simulink model "HW6_Q3_2slx_2021a"  (R2021a)
settings: Solver=VariableStepAuto  StartTime=0.0  StopTime=15.0  RelTol=1e-3
settings Model: Creator=USER  LastModifiedBy=USER
settings DebuggingCC: UnconnectedInputMsg=none  UnconnectedOutputMsg=none  UnconnectedLineMsg=none
settings ModelReferenceCC: EnableRefExpFcnMdlSchedulingChecks=off
settings RTWCC: Description=Generic Real-Time Target  DLArmComputeVersion=20.02.1

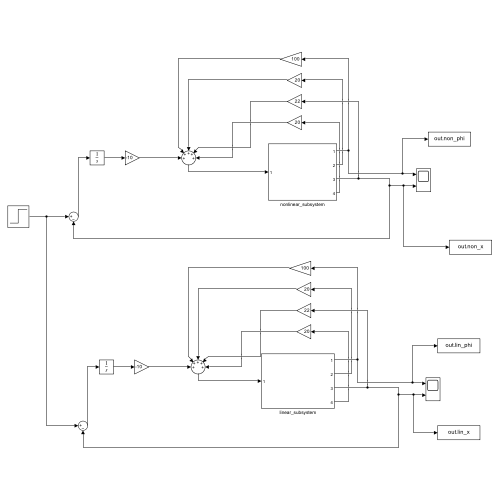
[thumbnail: Simulink's stored preview of the top-level diagram]
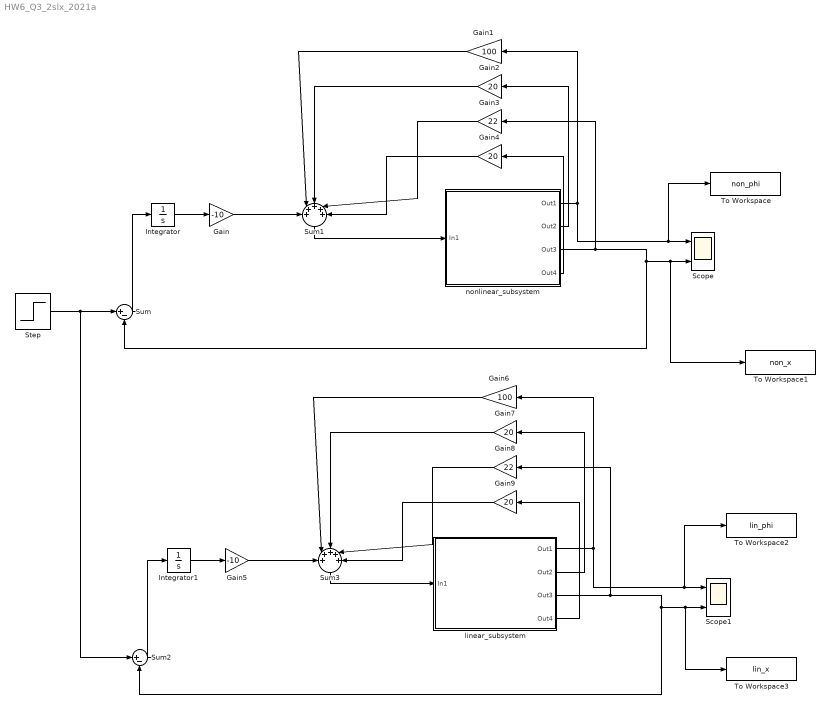
== system HW6_Q3_2slx_2021a ==
  Gain : Gain  Gain=-10
  Gain1 : Gain  Gain=100
  Gain{2,4,7,9} (4 alike) : Gain  Gain=20
  Gain3 : Gain  Gain=22
  Gain5 : Gain  Gain=-10
  Gain6 : Gain  Gain=100
  Gain8 : Gain  Gain=22
  Integrator : Integrator
  Integrator1 : Integrator
  Scope : Scope  NumInputPorts=2
  Scope1 : Scope  NumInputPorts=2
  Step : Step  Time=5  SampleTime=0
  Sum : Sum  Inputs=|+-
  Sum1 : Sum  Inputs=+++++
  Sum2 : Sum  Inputs=|+-
  Sum3 : Sum  Inputs=+++++
  To Workspace : ToWorkspace  VariableName=non_phi  SaveFormat=Timeseries  SampleTime=-1
  To Workspace1 : ToWorkspace  VariableName=non_x  SaveFormat=Timeseries  SampleTime=-1
  To Workspace2 : ToWorkspace  VariableName=lin_phi  SaveFormat=Timeseries  SampleTime=-1
  To Workspace3 : ToWorkspace  VariableName=lin_x  SaveFormat=Timeseries  SampleTime=-1
  linear_subsystem : Subsystem
  nonlinear_subsystem : Subsystem
  wires:
  nonlinear_subsystem/3(Out3) -> Gain3/1, Sum/2, To Workspace1/1, Scope/2
  Step/1 -> Sum2/1, Sum/1
  Sum/1 -> Integrator/1
  Sum1/1 -> nonlinear_subsystem/1(In1)
  Integrator/1 -> Gain/1
  Gain/1 -> Sum1/1
  nonlinear_subsystem/1(Out1) -> To Workspace/1, Scope/1, Gain1/1
  nonlinear_subsystem/2(Out2) -> Gain2/1
  nonlinear_subsystem/4(Out4) -> Gain4/1
  Gain4/1 -> Sum1/5
  Gain3/1 -> Sum1/4
  Gain2/1 -> Sum1/3
  Gain1/1 -> Sum1/2
  linear_subsystem/2(Out2) -> Gain7/1
  Gain9/1 -> Sum3/5
  linear_subsystem/3(Out3) -> Gain8/1, Sum2/2, To Workspace3/1, Scope1/2
  Gain7/1 -> Sum3/3
  linear_subsystem/4(Out4) -> Gain9/1
  linear_subsystem/1(Out1) -> To Workspace2/1, Scope1/1, Gain6/1
  Sum2/1 -> Integrator1/1
  Integrator1/1 -> Gain5/1
  Gain5/1 -> Sum3/1
  Gain6/1 -> Sum3/2
  Sum3/1 -> linear_subsystem/1(In1)
  Gain8/1 -> Sum3/4

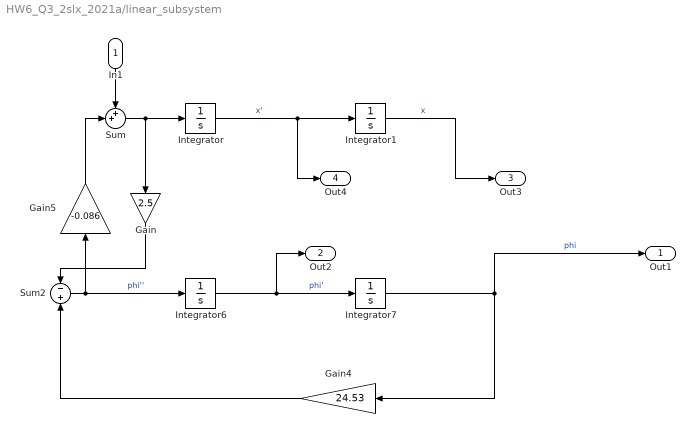
== system HW6_Q3_2slx_2021a/linear_subsystem ==
  In1 : Inport
  Gain : Gain  Gain=2.5
  Gain4 : Gain  Gain=24.53
  Gain5 : Gain  Gain=-0.086
  Integrator : Integrator
  Integrator1 : Integrator
  Integrator6 : Integrator
  Integrator7 : Integrator  InitialCondition=0.1
  Sum : Sum  Inputs=++|
  Sum2 : Sum  Inputs=-+
  Out1 : Outport
  Out2 : Outport  Port=2
  Out3 : Outport  Port=3
  Out4 : Outport  Port=4
  wires:
  Gain4/1 -> Sum2/2
  Integrator7/1 -> Out1/1, Gain4/1  "phi"
  Integrator1/1 -> Out3/1  "x"
  Integrator6/1 -> Out2/1, Integrator7/1  "phi'"
  Sum2/1 -> Integrator6/1, Gain5/1  "phi''"
  Integrator/1 -> Out4/1, Integrator1/1  "x'"
  Gain/1 -> Sum2/1
  In1/1 -> Sum/1
  Gain5/1 -> Sum/2
  Sum/1 -> Gain/1, Integrator/1

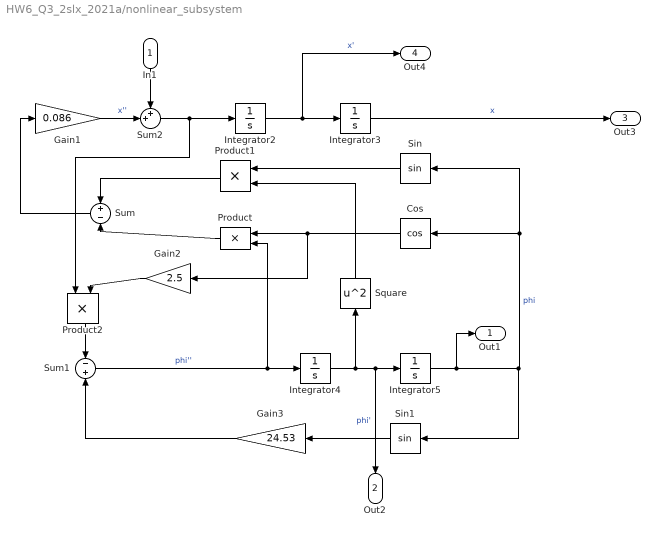
== system HW6_Q3_2slx_2021a/nonlinear_subsystem ==
  In1 : Inport
  Cos : Trigonometry  Operator=cos
  Gain1 : Gain  Gain=0.086
  Gain2 : Gain  Gain=2.5
  Gain3 : Gain  Gain=24.53
  Integrator2 : Integrator
  Integrator3 : Integrator
  Integrator4 : Integrator
  Integrator5 : Integrator  InitialCondition=0.1
  Product : Product
  Product1 : Product
  Product2 : Product
  Sin : Trigonometry
  Sin1 : Trigonometry
  Square : Math  Operator=square  SaturateOnIntegerOverflow=on
  Sum : Sum  Inputs=+-
  Sum1 : Sum  Inputs=-+
  Sum2 : Sum  Inputs=++|
  Out1 : Outport
  Out2 : Outport  Port=2
  Out3 : Outport  Port=3
  Out4 : Outport  Port=4
  wires:
  Product/1 -> Sum/2
  Product2/1 -> Sum1/1
  Gain2/1 -> Product2/2
  Integrator2/1 -> Out4/1, Integrator3/1  "x'"
  Integrator5/1 -> Out1/1, Sin/1, Cos/1, Sin1/1  "phi"
  Integrator3/1 -> Out3/1  "x"
  Sum1/1 -> Product/2, Integrator4/1  "phi''"
  Product1/1 -> Sum/1
  Cos/1 -> Gain2/1, Product/1
  Square/1 -> Product1/2
  Sin/1 -> Product1/1
  Sin1/1 -> Gain3/1
  Sum/1 -> Gain1/1
  Integrator4/1 -> Square/1, Out2/1, Integrator5/1  "phi'"
  Gain3/1 -> Sum1/2
  In1/1 -> Sum2/1
  Gain1/1 -> Sum2/2  "x''"
  Sum2/1 -> Product2/1, Integrator2/1
